simulink model "BUCK_ESO_SMC_08022311_R2022"  (R2022b)
settings: Solver=VariableStepAuto  StartTime=0.0  StopTime=3  RelTol=1e-3
values from neighbouring files (symbols this model uses):
  beta1 = 20    [BUCK_ESO_SMC_parameter_08022311.m]
  beta2 = 100    [BUCK_ESO_SMC_parameter_08022311.m]
  C0 = 0.001    [BUCK_ESO_SMC_parameter_08022311.m]
  eta = 100000    [BUCK_ESO_SMC_parameter_08022311.m]
  k = 1000    [BUCK_ESO_SMC_parameter_08022311.m]
  L0 = 0.01    [BUCK_ESO_SMC_parameter_08022311.m]
  R0 = 20    [BUCK_ESO_SMC_parameter_08022311.m]
  Rd = 2    [BUCK_ESO_SMC_parameter_08022311.m]
  Vin0 = 24    [BUCK_ESO_SMC_parameter_08022311.m]
  Vr = 10    [BUCK_ESO_SMC_parameter_08022311.m]
libraries: spsSeriesRLCBranchLib x4, spsMosfetLib x2, spsDiodeLib x1, simulink x1, spsVoltageMeasurementLib x1, spsDCVoltageSourceLib x1, spsCurrentMeasurementLib x1, spspowerguiLib x1
settings Model: Creator=ASUS  LastModifiedBy=ASUS
settings RTWCC: GPUComputeCapability=5.0

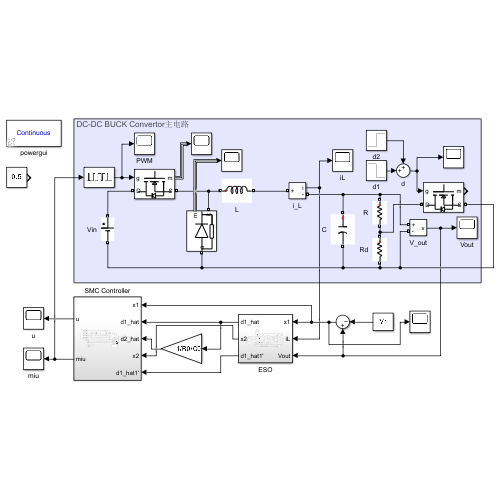
[thumbnail: Simulink's stored preview of the top-level diagram]
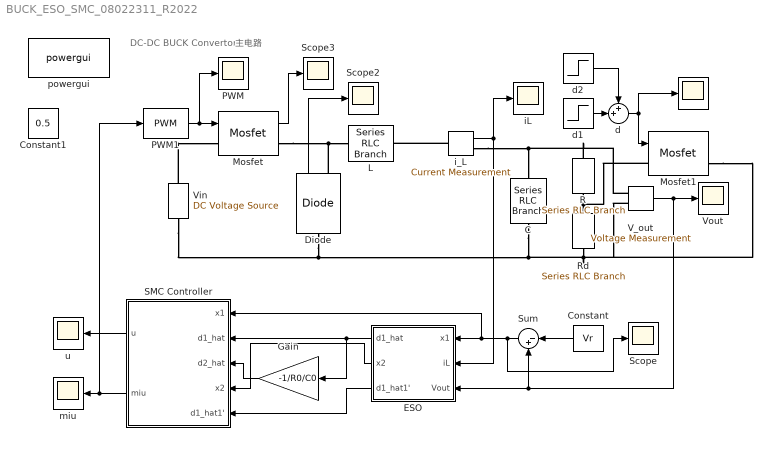
== system BUCK_ESO_SMC_08022311_R2022 ==
  note: DC-DC BUCK Convertor主电路
  " " : Scope
  C : spsSeriesRLCBranchLib/Series RLC Branch  LConnTagsString=__new0  RConnTagsString=__new0  BranchType=C  Resistance=1  Inductance=0.01  SetiL0=off  InitialCurrent=0  Capacitance=C0  Setx0=on  InitialVoltage=0  Measurements=None
  Constant : Constant  Value=Vr
  Constant1 : Constant  Value=0.5
  Diode : spsDiodeLib/Diode  Ron=0.001  Lon=0  Vf=0.8  IC=0  UseSnubber=0  Rs=500  Cs=250e-9  Measurements=on
  ESO : Subsystem
  Gain : Gain  Gain=-1/R0/C0
  L : spsSeriesRLCBranchLib/Series RLC Branch  LConnTagsString=__new0  RConnTagsString=__new0  BranchType=L  Resistance=1  Inductance=L0  SetiL0=off  InitialCurrent=0  Capacitance=1e-6  Setx0=off  InitialVoltage=0  Measurements=None
  Mosfet : spsMosfetLib/Mosfet  Ron=0.1  Lon=0  Rd=0.01  Vfd=0  IC=0  Rs=1e5  Cs=inf  Measurements=on
  Mosfet1 : spsMosfetLib/Mosfet  Ron=0.1  Lon=0  Rd=0.01  Vfd=0  IC=0  Rs=1e5  Cs=inf  Measurements=on
  PWM : Scope
  PWM1 : simulink/Discontinuities/PWM  DisableCoverage=on  Period=1/20e+3  InitialDelay=0  DisallowZeroDutyCycle=off  RunAtFixedTimeIntervals=off  SampleTime=0.1
  R : spsSeriesRLCBranchLib/Series RLC Branch  LConnTagsString=__new0  RConnTagsString=__new0  BranchType=R  Resistance=R0  Inductance=0.01  SetiL0=off  InitialCurrent=0  Capacitance=1e-3  Setx0=off  InitialVoltage=0  Measurements=None
  Rd : spsSeriesRLCBranchLib/Series RLC Branch  LConnTagsString=__new0  RConnTagsString=__new0  BranchType=R  Resistance=Rd  Inductance=0.01  SetiL0=off  InitialCurrent=0  Capacitance=1e-3  Setx0=off  InitialVoltage=0  Measurements=None
  SMC Controller : Subsystem
  Scope : Scope
  Scope2 : Scope
  Scope3 : Scope
  Sum : Sum  Inputs=|-+
  V_out : spsVoltageMeasurementLib/Voltage Measurement  PhasorSimulation=off  OutputType=Complex  PSBequivalent=0
  Vin : spsDCVoltageSourceLib/DC Voltage Source  Amplitude=Vin0  Measurements=None
  Vout : Scope
  d : Sum  Inputs=++|
  d1 : Step  Before=1  After=0  SampleTime=0
  d2 : Step  Time=2  SampleTime=0
  iL : Scope
  i_L : spsCurrentMeasurementLib/Current Measurement  PhasorSimulation=off  OutputType=Complex  PSBequivalent=0
  miu : Scope
  powergui : spspowerguiLib/powergui  Priority=1  SimulationMode=Continuous  SampleTime=50e-6  frequency=60  Iterations=50  frequencyindice=0  Pbase=100e6  ErrMax=1e-4  UnitsV=kV  UnitsW=MW  buscounter=0  FunctionMessages=off  echomessages=off  EnableUseOfTLC=off  CurrentSourceSwitches=off  DisableSnubberDevices=off  DisableRonSwitches=off  DisableVfSwitches=off  DisplayEquations=off  AutomaticDiscreteSolvers=off  SolverType=Tustin/Backward Euler (TBE)  Interpol=off  ExternalGateDelay=off  methode=off  Ts=100  x0status=blocks  SPID=on  SwTol=0  HookPort=off  NonlinearTolerance=1e-4  nMaxIteration=100  ContinueOnMaxIteration=off  RestoreLinks=warning  ResistiveCurrentMeasurement=off  Frange=[0:2:500]  Ylog=off  Xlog=on  ShowGrid=off  save=off  variable=ZData  structure=0  ZoomFFT=off  StartTime=0.0  cycles=1  DisplayStyle=1  fundamental=60  FreqAxis=off  MaxFrequency=1000  frequencyindicesteady=1  RmsSteady=1  display=off
  u : Scope
  wires:
  i_L/1 -> ESO/2(iL), iL/1
  Diode/1 -> Scope2/1
  Mosfet/1 -> Scope3/1
  ESO/1(d1_hat) -> Gain/1, SMC Controller/2(d1_hat)
  Gain/1 -> SMC Controller/3(d2_hat)
  Sum/1 -> Scope/1, SMC Controller/1(x1), ESO/1(x1)
  SMC Controller/1(u) -> u/1
  PWM1/1 -> PWM/1, Mosfet/1
  ESO/2(x2) -> SMC Controller/4(x2)
  SMC Controller/2(miu) -> PWM1/1, miu/1
  ESO/3(d1_hat1') -> SMC Controller/5(d1_hat1')
  Constant/1 -> Sum/1
  V_out/1 -> Sum/2, ESO/3(Vout), Vout/1
  d1/1 -> d/2
  d2/1 -> d/1
  d/1 -> " "/1, Mosfet1/1
  connections:
  Vin/RConn1 -- Mosfet/LConn1
  Mosfet/RConn1 -- Diode/RConn1 -- L/LConn1
  i_L/LConn1 -- L/RConn1
  i_L/RConn1 -- V_out/LConn1 -- R/LConn1 -- C/LConn1
  Diode/LConn1 -- Vin/LConn1 -- Mosfet1/RConn1 -- V_out/LConn2 -- Rd/RConn1 -- C/RConn1
  Rd/LConn1 -- Mosfet1/LConn1 -- R/RConn1

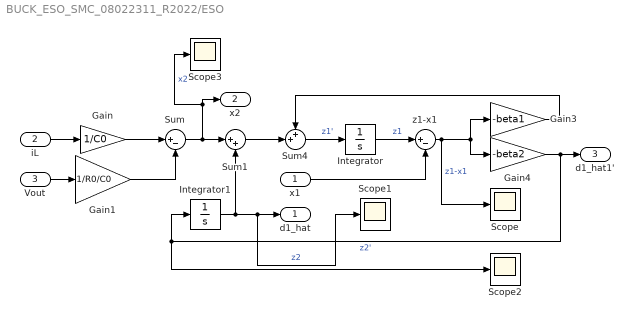
== system BUCK_ESO_SMC_08022311_R2022/ESO ==
  x1 : Inport
  iL : Inport  Port=2
  Vout : Inport  Port=3
  Gain : Gain  Gain=1/C0
  Gain1 : Gain  Gain=1/R0/C0
  Gain3 : Gain  Gain=-beta1
  Gain4 : Gain  Gain=-beta2
  Integrator : Integrator
  Integrator1 : Integrator
  Scope{,1..3} (4 alike) : Scope
  Sum : Sum  Inputs=|+-
  Sum1 : Sum  Inputs=|++
  Sum4 : Sum  Inputs=++|
  z1-x1 : Sum  Inputs=|+-
  d1_hat : Outport
  x2 : Outport  Port=2
  d1_hat1' : Outport  Port=3
  wires:
  Vout/1 -> Gain1/1
  iL/1 -> Gain/1
  Gain1/1 -> Sum/2
  Gain/1 -> Sum/1
  Integrator1/1 -> Sum1/2, Scope1/1, d1_hat/1  "z2"
  Sum/1 -> Scope3/1, x2/1, Sum1/1  "x2"
  Sum4/1 -> Integrator/1  "z1'"
  x1/1 -> z1-x1/2
  Sum1/1 -> Sum4/2
  Gain3/1 -> Sum4/1
  Gain4/1 -> Integrator1/1, Scope2/1, d1_hat1'/1  "z2'"
  Integrator/1 -> z1-x1/1  "z1"
  z1-x1/1 -> Scope/1, Gain4/1, Gain3/1  "z1-x1"

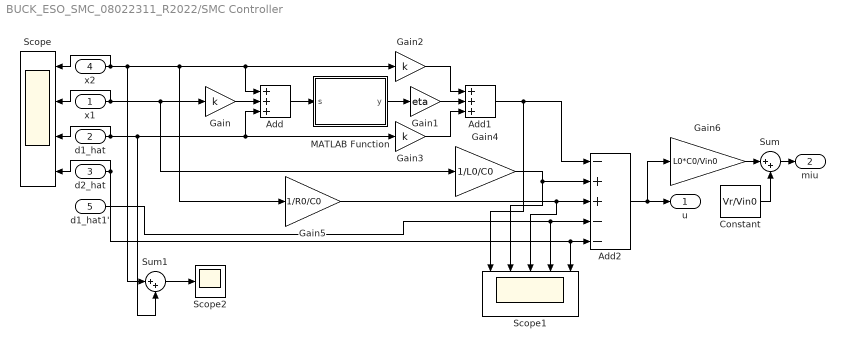
== system BUCK_ESO_SMC_08022311_R2022/SMC Controller ==
  x1 : Inport
  d1_hat : Inport  Port=2
  d2_hat : Inport  Port=3
  x2 : Inport  Port=4
  d1_hat1' : Inport  Port=5
  Add : Sum  Inputs=+++
  Add1 : Sum  Inputs=+++
  Add2 : Sum  Inputs=-++--
  Constant : Constant  Value=Vr/Vin0
  Gain : Gain  Gain=k
  Gain1 : Gain  Gain=eta
  Gain2 : Gain  Gain=k
  Gain3 : Gain  Gain=k
  Gain4 : Gain  Gain=1/L0/C0
  Gain5 : Gain  Gain=1/R0/C0
  Gain6 : Gain  Gain=L0*C0/Vin0
  MATLAB Function : MATLAB Function  TreatAsAtomicUnit=on
  Scope : Scope  NumInputPorts=4
  Scope1 : Scope  NumInputPorts=5
  Scope2 : Scope
  Sum : Sum  Inputs=|++
  Sum1 : Sum  Inputs=|++
  u : Outport
  miu : Outport  Port=2
  wires:
  x1/1 -> Scope/2, Gain/1, Gain4/1
  Gain/1 -> Add/2
  x2/1 -> Scope/1, Gain5/1, Add/1, Gain2/1, Sum1/1
  d1_hat/1 -> Scope/3, Sum1/2, Gain3/1, Add/3
  Add/1 -> MATLAB Function/1(s)
  MATLAB Function/1(y) -> Gain1/1
  Gain1/1 -> Add1/2
  Gain2/1 -> Add1/1
  Gain3/1 -> Add1/3
  Gain4/1 -> Scope1/2, Add2/2
  Gain5/1 -> Scope1/3, Add2/3
  d2_hat/1 -> Scope/4, Scope1/5, Add2/5
  Add1/1 -> Scope1/1, Add2/1
  Add2/1 -> Gain6/1, u/1
  Gain6/1 -> Sum/1
  Sum/1 -> miu/1
  Constant/1 -> Sum/2
  d1_hat1'/1 -> Scope1/4, Add2/4
  Sum1/1 -> Scope2/1

== matlab function BUCK_ESO_SMC_08022311_R2022/SMC Controller/MATLAB Function ==
  data: s input; y output
function y = sgn(s)
    if s > 0
        y = 1;
    elseif s < 0
        y = -1;
    else
        y = 0;
    end
end
